simulink model "pole_placement_with_disturbance"  (R2023b)
settings: Solver=FixedStepAuto  StartTime=0.0  StopTime=Tend_slk  RelTol=1e-3
values from neighbouring files (symbols this model uses):
  Kv = [-1.64697547352e-05  2.12268535147e-05  1.88764310292e-05; 2.30722124708e-05  -3.65669674193e-05  -3.23919550811e-05; 3.25171076399e-05  -5.05969618035e-05  -5.1583153022e-05]    [K_pole_robust.mat]    (also in K_pole_slow.mat = [-1.41162623643e-05  3.15575037387e-07  3.72300385462e-06; 6; K_pole_slow1.mat = [-2.53659790778e-06  1.31318924073e-06  5.41586357513e-07; 1; main_pole.m = K(:,7:9))
  Kx = [0.000682996894791 0.0374777376708 -6.3928150212e-05 0.0375333008063 0.00147412825874 0.00310964805818 -0.000671461003357 0.00114998106287 0.00196075496481 0.00715176146332 -0.00705310314004 -0.0100224248261 ... (18 elements, 3x6)]    [K_pole_robust.mat]    (also in K_pole_slow.mat = [0.000507417558982 -1.92491548473e-05 -0.000125814013907 -1.; K_pole_slow1.mat = [0.00015515456069 0.0383006342581 0.0011252624163 0.03830904; main_pole.m = K(:,1:6))
  param = [Ixx;Iyy;Izz;l;k;b;m]    [main_pole.m]
  Ts_slk = 0.01    [main_pole.m]
  x0 = [1;1;1;0;0;0]*0.01    [main_pole.m]
  x_des = [1;1;1;0;0;0]    [main_pole.m]
libraries: SignalEditorBlockLib x1
settings Model: Creator=asus  LastModifiedBy=asus
settings OptimizationCC: ReuseModelBlockBuffer=off

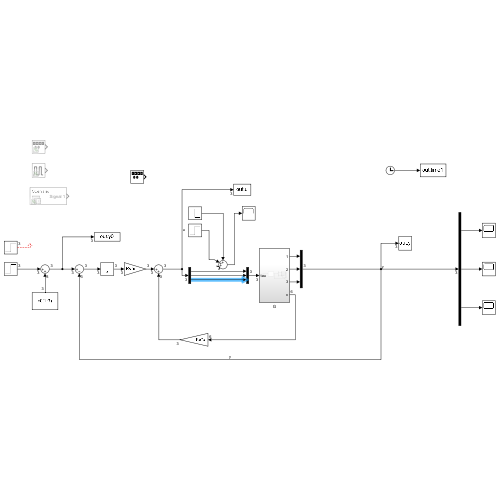
[thumbnail: Simulink's stored preview of the top-level diagram]
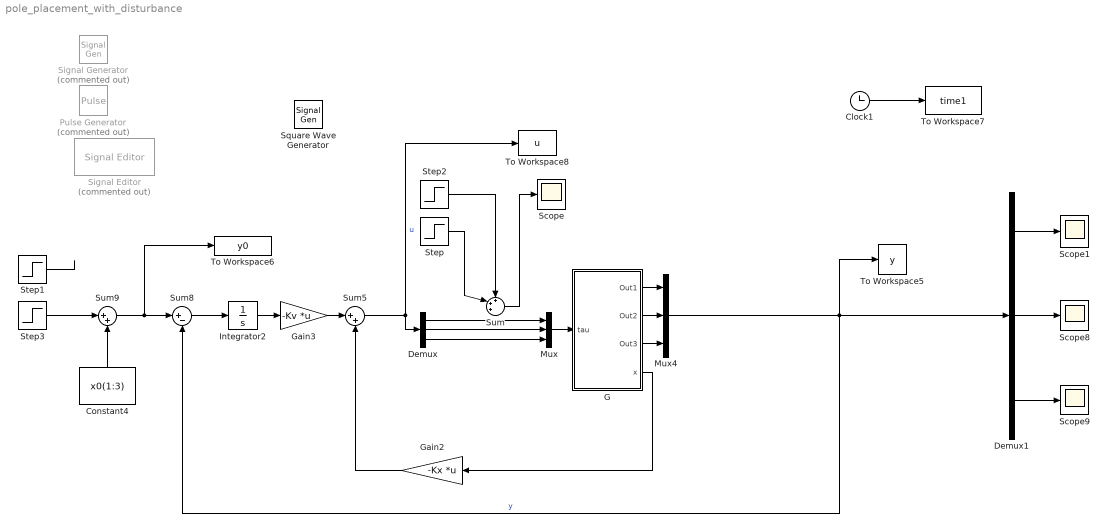
== system pole_placement_with_disturbance ==
  Clock1 : Clock
  Constant4 : Constant  Value=x0(1:3)
  Demux : Demux  Outputs=3
  Demux1 : Demux  Outputs=3
  G : Subsystem
  Gain2 : Gain  Gain=-Kx  Multiplication=Matrix(K*u)
  Gain3 : Gain  Gain=-Kv  Multiplication=Matrix(K*u)
  Integrator2 : Integrator
  Mux : Mux  Inputs=3
  Mux4 : Mux  Inputs=3
  Pulse Generator : DiscretePulseGenerator  Commented=on  PulseType=Time based  Amplitude=0.1  Period=0.5  PulseWidth=5
  Scope{,1,8..9} (4 alike) : Scope
  Signal Generator : SignalGenerator  Commented=on  WaveForm=square  Amplitude=0.1  Frequency=2  Units=rad/sec
  Signal Editor : SignalEditorBlockLib/Signal Editor  Commented=on  FileName=untitled.mat  ActiveScenario=Scenario  ActiveSignal=Signal 1  IsBus=off  OutputBusObjectStr=Bus: BusObject  SampleTime=0  Interpolate=off  ZeroCross=off  OutputAfterFinalValue=Setting to zero  Unit=inherit  PreserveSignalName=on  ApplySigPropsToAllScenarios=on  ApplySigPropsToAllSignals=off
  Square Wave Generator : SignalGenerator  WaveForm=square  Units=rad/sec
  Step : Step  Time=200  After=0.1  SampleTime=Ts_slk
  Step1 : Step  Time=0  After=x_des(1:3)*30*pi/180*0  SampleTime=0
  Step2 : Step  Time=200.1  Before=0.1  After=0  SampleTime=Ts_slk
  Step3 : Step  Time=0  After=[0.5;0.5;0.5]*0  SampleTime=0
  Sum : Sum  Inputs=+++|
  Sum5 : Sum  Inputs=|++
  Sum8 : Sum  Inputs=|+-
  Sum9 : Sum  Inputs=|++
  To Workspace5 : ToWorkspace  VariableName=y  SampleTime=-1
      settings: Save2DSignal=2-D array (concatenate along first dimension)
  To Workspace6 : ToWorkspace  VariableName=y0  SampleTime=Ts_slk
  To Workspace7 : ToWorkspace  VariableName=time1  SampleTime=Ts_slk
      settings: Save2DSignal=2-D array (concatenate along first dimension)
  To Workspace8 : ToWorkspace  VariableName=u  SampleTime=Ts_slk
  wires:
  Mux4/1 -> Demux1/1, Sum8/2, To Workspace5/1  "y"
  Sum8/1 -> Integrator2/1
  Gain2/1 -> Sum5/2
  Demux1/2 -> Scope8/1
  Gain3/1 -> Sum5/1
  Sum9/1 -> To Workspace6/1, Sum8/1
  Sum5/1 -> To Workspace8/1, Demux/1  "u"
  Constant4/1 -> Sum9/2
  Clock1/1 -> To Workspace7/1
  Demux1/3 -> Scope9/1
  Integrator2/1 -> Gain3/1
  Step1/1 -> ?
  Demux1/1 -> Scope1/1
  G/1(Out1) -> Mux4/1
  G/3(Out3) -> Mux4/3
  G/2(Out2) -> Mux4/2
  G/4(x) -> Gain2/1
  Sum/1 -> Scope/1
  Demux/1 -> Mux/1
  Demux/2 -> Mux/2
  Mux/1 -> G/1("tau ")
  Demux/3 -> Mux/3
  Step/1 -> Sum/2
  Step2/1 -> Sum/1
  Step3/1 -> Sum9/1

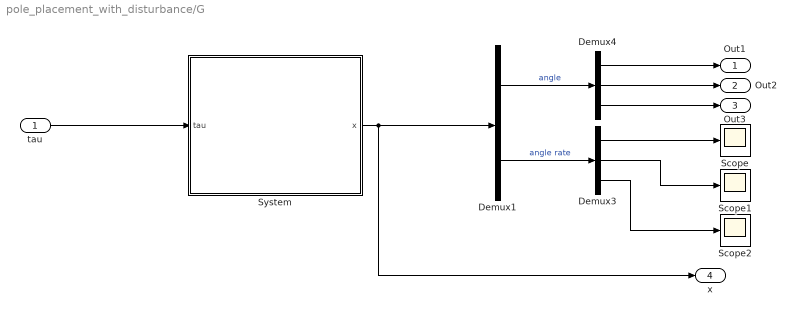
== system pole_placement_with_disturbance/G ==
  "tau " : Inport
  Demux1 : Demux  Outputs=2
  Demux3 : Demux  Outputs=3
  Demux4 : Demux  Outputs=3
  Scope : Scope
  Scope1 : Scope
  Scope2 : Scope
  System : Subsystem
  Out1 : Outport
  Out2 : Outport  Port=2
  Out3 : Outport  Port=3
  x : Outport  Port=4
  wires:
  Demux4/3 -> Out3/1
  System/1(x) -> x/1, Demux1/1
  Demux3/1 -> Scope/1
  Demux4/1 -> Out1/1
  Demux1/1 -> Demux4/1  "angle"
  Demux1/2 -> Demux3/1  "angle rate"
  Demux3/2 -> Scope1/1
  Demux4/2 -> Out2/1
  "tau "/1 -> System/1("tau ")
  Demux3/3 -> Scope2/1

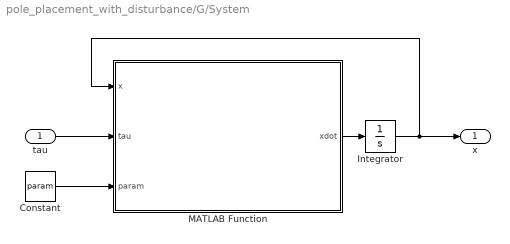
== system pole_placement_with_disturbance/G/System ==
  "tau " : Inport
  Constant : Constant  Value=param
  Integrator : Integrator  InitialCondition=x0
  MATLAB Function : MATLAB Function  TreatAsAtomicUnit=on
  x : Outport
  wires:
  Integrator/1 -> MATLAB Function/1(x), x/1
  MATLAB Function/1(xdot) -> Integrator/1
  "tau "/1 -> MATLAB Function/2(tau)
  Constant/1 -> MATLAB Function/3(param)

== matlab function pole_placement_with_disturbance/G/System/MATLAB Function ==
  data: x input; tau input; xdot output; param input
function xdot =quadcopter(x,tau,param)
% Inputs:
%           x       (model state)
%           tau     (torque)           
%           param   (model parameters)
%
% Outputs:  x_dot  (derivative of the state with respect to time)

% Parameters
g        =       9.81;           %  gravity acceleration (m/s^2)
Ixx      =       param(1,1);     %  moment of inertia 
Iyy      =       param(2,1);     %  moment of inertia
Izz      =       param(3,1);     %  moment of inertia 

% States
phi      =       x(1,1);     %  roll angle (rad)
theta    =       x(2,1);     %  pitch angle (rad)
psi      =       x(3,1);     %  yaw angle (rad)  
phi_dot  =       x(4,1);     %  roll rate (rad/s)
theta_dot=       x(5,1);     %  pitch rate (rad/s)
psi_dot  =       x(6,1);     %  yaw rate (rad/s)  

cph         =       cos(phi);
cth         =       cos(theta);
cps         =       cos(psi);
sph         =       sin(phi);
sth         =       sin(theta);
sps         =       sin(psi);

% torques
tau_1    =       tau(1,1);   %  roll torque 
tau_2    =       tau(2,1);   %  pitch torque 
tau_3    =       tau(3,1);   %  yaw torque   

% Coriolis matrix
C11=  0;
C12= (Iyy-Izz)*(theta_dot*cph*sph+psi_dot*sph^2*cth)+(Izz-Iyy)*psi_dot*cph^2*cth-Ixx*psi_dot*cth;
C13= (Izz-Iyy)*psi_dot*cph*sph*cth^2;
C21= (Izz-Iyy)*(theta_dot*cph*sph+psi_dot*sph*cth)+(Iyy-Izz)*psi_dot*cph^2*cth+Ixx*psi_dot*cth;
C22= (Izz-Iyy)*psi_dot*cph*sph;
C23= -Ixx*psi_dot*sth*cth+Iyy*psi_dot*sph^2*sth*cth+Izz*psi_dot*cph^2*sth*cth;
C31= (Iyy-Izz)*psi_dot*cth^2*sph*cph-Ixx*theta_dot*cth;
C32= (Izz-Iyy)*(theta_dot*cph*sph*sth+phi_dot*sph^2*cth)+(Iyy-Izz)*phi_dot*cph^2*cth+Ixx*psi_dot*sth*cth-Iyy*psi_dot*sph^2*sth*cth-Izz*psi_dot*cph^2*sth*cth;
C33= (Iyy-Izz)*phi_dot*cph*sph*cth^2-Iyy*theta_dot*sph^2*cth*sth-Izz*theta_dot*cph^2*cth*sth+Ixx*theta_dot*cth*sth;

C  = [C11 C12 C13;
    C21 C22 C23;
    C31 C32 C33];

% Inertia matrix
J11= Ixx;
J12= 0;
J13= -Ixx*sth;
J21= 0;
J22= Iyy*cph^2+Izz*sph^2;
J23= (Iyy-Izz)*cph*sph*cth;
J31= -Ixx*sth;
J32= (Iyy-Izz)*cph*sph*cth;
J33= Ixx*sth^2+Iyy*sph^2*cth^2+Izz*cph^2*cth^2;

J  = [J11 J12 J13;
    J21 J22 J23;
    J31 J32 J33];
v_wind = 2;
Cdz    = 0.176;
R      = 0.08;
Az     = 4*pi*R^2;
rho    = 1.204;
Fdz    =-1/2*rho*Cdz*Az*v_wind^2*sign(v_wind);
Fd     = [0;0;Fdz];
%% Model Equation 
invJ = [ (J22*J33 - J23*J32)/(J11*J22*J33 - J11*J23*J32 - J12*J21*J33 + J12*J23*J31 + J13*J21*J32 - J13*J22*J31), -(J12*J33 - J13*J32)/(J11*J22*J33 - J11*J23*J32 - J12*J21*J33 + J12*J23*J31 + J13*J21*J32 - J13*J22*J31),  (J12*J23 - J13*J22)/(J11*J22*J33 - J11*J23*J32 - J12*J21*J33 + J12*J23*J31 + J13*J21*J32 - J13*J22*J31);
         -(J21*J33 - J23*J31)/(J11*J22*J33 - J11*J23*J32 - J12*J21*J33 + J12*J23*J31 + J13*J21*J32 - J13*J22*J31),  (J11*J33 - J13*J31)/(J11*J22*J33 - J11*J23*J32 - J12*J21*J33 + J12*J23*J31 + J13*J21*J32 - J13*J22*J31), -(J11*J23 - J13*J21)/(J11*J22*J33 - J11*J23*J32 - J12*J21*J33 + J12*J23*J31 + J13*J21*J32 - J13*J22*J31);
         (J21*J32 - J22*J31)/(J11*J22*J33 - J11*J23*J32 - J12*J21*J33 + J12*J23*J31 + J13*J21*J32 - J13*J22*J31), -(J11*J32 - J12*J31)/(J11*J22*J33 - J11*J23*J32 - J12*J21*J33 + J12*J23*J31 + J13*J21*J32 - J13*J22*J31),  (J11*J22 - J12*J21)/(J11*J22*J33 - J11*J23*J32 - J12*J21*J33 + J12*J23*J31 + J13*J21*J32 - J13*J22*J31);];

xdot        = zeros(6,1);
xdot(1:3,1) = x(4:6,1);
xdot(4:6,1) = invJ*(tau - Fd - C*x(4:6,1));
